simulink model "Teste_VSI"  (R2015a)
settings: Solver=ode45  StartTime=0.0  StopTime=0.05  MaxStep=1e-5  RelTol=1e-3
libraries: powerlib x10, AvgModels x1, powerlib_meascontrol x1, simulink x1
settings Model: CovSFcnEnable=off  Creator=lgalotto  LastModifiedBy=lgalo
settings DebuggingCC: SolverPrmCheckMsg=warning  UnconnectedInputMsg=none  UnconnectedOutputMsg=none  UnconnectedLineMsg=none

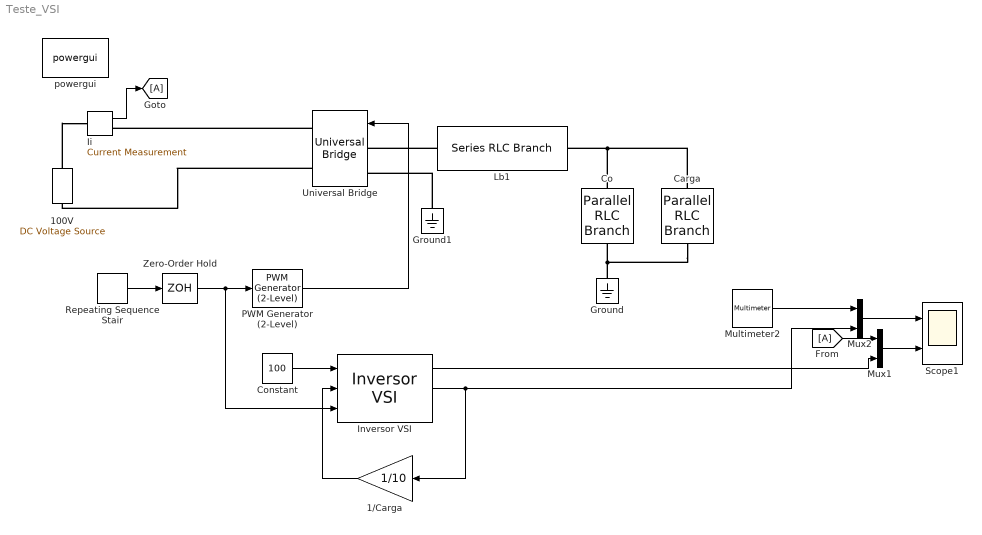
== system Teste_VSI ==
  1/Carga : Gain  Gain=1/10
  100V : powerlib/Electrical Sources/DC Voltage Source  Amplitude=100  Measurements=None
  Carga : powerlib/Elements/Parallel RLC Branch  LConnTagsString=a  RConnTagsString=__new0  BranchType=R  Resistance=10  Inductance=1e-3  SetiL0=off  InitialCurrent=0  Capacitance=100e-6  Setx0=off  InitialVoltage=0  Measurements=Branch voltage
  Co : powerlib/Elements/Parallel RLC Branch  LConnTagsString=a  RConnTagsString=__new0  BranchType=C  Resistance=10e3  Inductance=1e-3  SetiL0=off  InitialCurrent=0  Capacitance=100e-6  Setx0=on  InitialVoltage=0  Measurements=Branch voltage
  Constant : Constant  Value=100
  Ground : powerlib/Elements/Ground  LConnTagsString=a
  Ground1 : powerlib/Elements/Ground  LConnTagsString=a
  Ii : powerlib/Measurements/Current Measurement  PhasorSimulation=off  OutputType=Complex  PSBequivalent=0
  Inversor VSI : AvgModels/Conversores Eletrônicos de Potência/Inversor VSI  Lb=280e-6  Co=100e-6  ILb=0  Vco=0
  Lb1 : powerlib/Elements/Series RLC Branch  LConnTagsString=__new0  RConnTagsString=__new0  BranchType=RL  Resistance=1e-3  Inductance=280e-6  SetiL0=on  InitialCurrent=0  Capacitance=1e-6  Setx0=off  InitialVoltage=0  Measurements=Branch current
  Multimeter2 : powerlib/Measurements/Multimeter  PhasorSimulation=off  OutputType=Complex  sel=2  L=3  Gain=1  yselected={'Ub: Co'};  PSBOutputType=1  PSBequivalent=0  AxesSetting=[0,0.1,-100,100]  Display=0  SavedBlockNames=-11
  Mux1 : Mux  Inputs=2
  Mux2 : Mux  Inputs=2
  PWM Generator (2-Level) : powerlib_meascontrol/Pulse & Signal Generators/PWM Generator (2-Level)  ModulatorType=Single-phase full-bridge (4 pulses)  ModulatorMode=Unsynchronized  Fc=20000  Pc=90  nF=27  MinMax="[ -1  1 ]"  SamplingTechnique=Natural  ModulatingSignals=off  m=0.8  Freq=60  Phase=0  Ts=0  ShowCarrierOutport=off
  Repeating Sequence Stair : simulink/Sources/Repeating Sequence Stair  OutValues=[0.2 0.4 0.6 0.8 -0.6 -0.2].'  tsamp=0.01  OutMin=[]  OutMax=[]  OutDataTypeStr=double  OutputDataTypeScalingMode=double  OutDataType=fixdt(0,8)  ConRadixGroup=Best Precision: Vector-wise  OutScaling=2^-12
  Scope1 : Scope  NumInputPorts=2
      settings: TimeRange=0.05  YMin=-200~-60  YMax=100~80
  Universal Bridge : powerlib/Power Electronics/Universal Bridge  Arms=2  SnubberResistance=1e5  SnubberCapacitance=inf  Device=MOSFET / Diodes  Ron=1e-3  Lon=0  ForwardVoltages="[  0  0  ]"  ForwardVoltage=0  GTOparameters=[ 10e-6 , 20e-6 ]  IGBTparameters=[ 1e-6 , 2e-6 ]  Measurements=None  Measurements_2=None  converterType=Rectifier
  Zero-Order Hold : ZeroOrderHold  SampleTime=0.01
  powergui : powerlib/powergui  Priority=1  SimulationMode=Continuous  SolverType=Tustin  SampleTime=50e-6  frequency=60  SPID=on  DisableSnubberDevices=off  DisableRonSwitches=off  DisableVfSwitches=off  SwTol=0  DisplayEquations=off  Interpol=off  methode=off  Ts=0  FunctionMessages=off  echomessages=off  HookPort=off  EnableUseOfTLC=off  x0status=blocks  frequencyindice=0  Pbase=100e6  ErrMax=1e-4  Iterations=50  UnitsV=kV  UnitsW=MW  buscounter=0  RestoreLinks=warning  ResistiveCurrentMeasurement=off  Frange=[0:2:500]  Ylog=off  Xlog=on  ShowGrid=off  save=off  variable=ZData  structure=0  ZoomFFT=off  StartTime=0.0  cycles=1  DisplayStyle=1  fundamental=60  FreqAxis=off  MaxFrequency=1000  frequencyindicesteady=1  RmsSteady=1  display=off
  wires:
  [A] -> Mux1/1
  Ii/1 -> [A]
  Constant/1 -> Inversor VSI/1
  Multimeter2/1 -> Mux2/1
  Inversor VSI/2 -> 1/Carga/1, Mux2/2
  Inversor VSI/1 -> Mux1/2
  Mux1/1 -> Scope1/2
  Mux2/1 -> Scope1/1
  Repeating Sequence Stair/1 -> Zero-Order Hold/1
  PWM Generator (2-Level)/1 -> Universal Bridge/1
  Zero-Order Hold/1 -> Inversor VSI/3, PWM Generator (2-Level)/1
  1/Carga/1 -> Inversor VSI/2
  connections:
  Co/LConn1 -- Lb1/RConn1 -- Carga/LConn1
  Ground/LConn1 -- Carga/RConn1 -- Co/RConn1
  100V/RConn1 -- Ii/LConn1
  Ground1/LConn1 -- Universal Bridge/LConn2
  Lb1/LConn1 -- Universal Bridge/LConn1
  Universal Bridge/RConn2 -- 100V/LConn1
  Universal Bridge/RConn1 -- Ii/RConn1
